simulink model "task_2_sim"  (R2023a)
settings: Solver=VariableStepAuto  StartTime=0.0  StopTime=2  MaxStep=0.00001  RelTol=1e-5
undefined symbols (not defined in the file): A, B, C, K, L, x0, x1
settings Model: Creator=user  LastModifiedBy=user

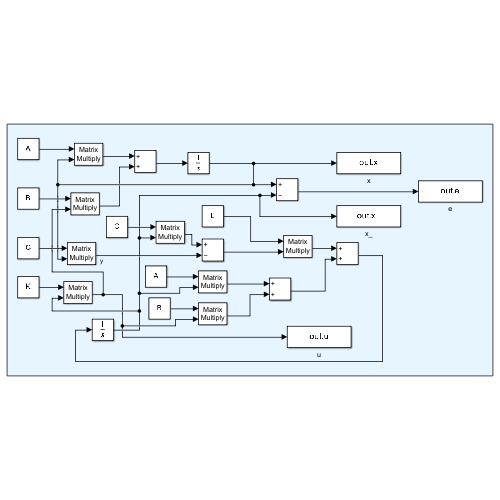
[thumbnail: Simulink's stored preview of the top-level diagram]
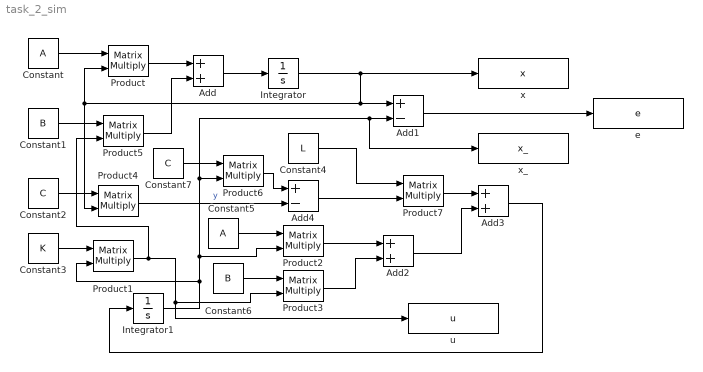
== system task_2_sim ==
  Add : Sum
  Add1 : Sum  Inputs=+-
  Add2 : Sum
  Add3 : Sum
  Add4 : Sum  Inputs=+-
  Constant : Constant  Value=A
  Constant1 : Constant  Value=B  VectorParams1D=off
  Constant2 : Constant  Value=C
  Constant3 : Constant  Value=K  VectorParams1D=off
  Constant4 : Constant  Value=L
  Constant5 : Constant  Value=A
  Constant6 : Constant  Value=B  VectorParams1D=off
  Constant7 : Constant  Value=C
  Integrator : Integrator  InitialCondition=x0
  Integrator1 : Integrator  InitialCondition=x1
  Product{,1..7} (8 alike) : Product  Multiplication=Matrix(*)
  e : ToWorkspace  VariableName=e  SaveFormat=Timeseries  SampleTime=-1
  u : ToWorkspace  VariableName=u  SaveFormat=Timeseries  SampleTime=-1
  x : ToWorkspace  VariableName=x  SaveFormat=Timeseries  SampleTime=-1
  x_ : ToWorkspace  VariableName=x_  SaveFormat=Timeseries  SampleTime=-1
  wires:
  Add/1 -> Integrator/1
  Constant/1 -> Product/1
  Product/1 -> Add/1
  Integrator/1 -> x/1, Product/2, Product4/2, Add1/1
  Constant1/1 -> Product5/1
  Product5/1 -> Add/2
  Add1/1 -> e/1
  Constant3/1 -> Product1/1
  Integrator1/1 -> Product6/2, x_/1, Add1/2, Product2/2, Product1/2
  Constant2/1 -> Product4/1
  Product4/1 -> Add4/2  "y"
  Constant5/1 -> Product2/1
  Product2/1 -> Add2/1
  Constant6/1 -> Product3/1
  Constant7/1 -> Product6/1
  Product6/1 -> Add4/1
  Add4/1 -> Product7/2
  Constant4/1 -> Product7/1
  Add3/1 -> Integrator1/1
  Product3/1 -> Add2/2
  Product1/1 -> Product5/2, Product3/2, u/1
  Product7/1 -> Add3/1
  Add2/1 -> Add3/2
